simulink model "ProyectoAutomatasSimulink_jona"  (R2015a)
settings: Solver=ode3  SolverMode=SingleTasking  StartTime=0.0  StopTime=inf  FixedStep=dt/10  RelTol=1e-3
values from neighbouring files (symbols this model uses):
  amaxh = 1    [ProyectoAutomatas.m]
  amaxt = 1    [ProyectoAutomatas.m]
  bah = Mh*nh*wposh    (= 69120)    [ProyectoAutomatas.m]
  bat = Mt*nt*wpost    (= 64800)    [ProyectoAutomatas.m]
  bh = beqh*rh^2/Rd^2    (= 28800)    [ProyectoAutomatas.m]
  bt = beqc*rc^2/Rw^2    (= 27000)    [ProyectoAutomatas.m]
  bw = 30*10^3    (= 30000)    [ProyectoAutomatas.m]
  distanciaSegMaxCarro = geometria.xt_max-constSegCarro    [ProyectoAutomatas.m]
  distanciaSegMinCarro = geometria.xt_min+constSegCarro    [ProyectoAutomatas.m]
  dt = 0.01    [ProyectoAutomatas.m]
  g = 9.80665    [ProyectoAutomatas.m]
  Kisah = Mh*wposh^3    (= 17905.2918847)    [ProyectoAutomatas.m]
  Kisat = Mt*wpost^3    (= 9768.17070431)    [ProyectoAutomatas.m]
  Ksah = Mh*nh*wposh^2    (= 49751.6587678)    [ProyectoAutomatas.m]
  Ksat = Mt*nt*wpost^2    (= 35580.2603037)    [ProyectoAutomatas.m]
  Kw = 1800*10^3    (= 1800000)    [ProyectoAutomatas.m]
  l_max_cable = 65    [ProyectoAutomatas.m]
  l_max_max_cable = 66    [ProyectoAutomatas.m]
  l_min_cable = 5    [ProyectoAutomatas.m]
  l_min_min_cable = 4    [ProyectoAutomatas.m]
  lh0 = 5    [ProyectoAutomatas.m]
  longitudSegMaxCable = l_max_cable-constSegCable    (= 60)    [ProyectoAutomatas.m]
  longitudSegMinCable = l_min_cable+constSegCable    (= 10)    [ProyectoAutomatas.m]
  mc = 50000    [ProyectoAutomatas.m]
  Mh = (Jdh+Jmh*rh^2) / (Rd^2)    (= 48014.2222222)    [ProyectoAutomatas.m]
  ml0 = 15000    [ProyectoAutomatas.m]
  mlfull = 65000    [ProyectoAutomatas.m]
  Mt = mc+(Jwc+Jmc*rc^2)/Rw^2    (= 59008)    [ProyectoAutomatas.m]
  na = 3    [ProyectoAutomatas.m]
  rc = 15    [ProyectoAutomatas.m]
  Rd = 0.75    [ProyectoAutomatas.m]
  rh = 30    [ProyectoAutomatas.m]
  Rw = 0.5    [ProyectoAutomatas.m]
  vh0 = 0    [ProyectoAutomatas.m]
  vlx0 = 0    [ProyectoAutomatas.m]
  vly0 = 0    [ProyectoAutomatas.m]
  vmaxh = 3    [ProyectoAutomatas.m]
  vmaxhfull = 1.5    [ProyectoAutomatas.m]
  vmaxhSobrepeso = 0.1    [ProyectoAutomatas.m]
  vmaxt = 4    [ProyectoAutomatas.m]
  vt0 = 0    [ProyectoAutomatas.m]
  xl0 = -30    [ProyectoAutomatas.m]
  xt0 = -30    [ProyectoAutomatas.m]
  xt_max = 50    [ParametrosGUIyTrayectoria.m]    (also in ProyectoAutomatas.m)
  xt_max_max = 51    [ParametrosGUIyTrayectoria.m]    (also in ProyectoAutomatas.m)
  xt_min = -30    [ParametrosGUIyTrayectoria.m]    (also in ProyectoAutomatas.m)
  xt_min_min = -31    [ParametrosGUIyTrayectoria.m]    (also in ProyectoAutomatas.m)
  yl0 = yt0-lh0-ml0*g/Kw    (= 39.9182779167)    [ProyectoAutomatas.m]
  yt0 = 45    [ProyectoAutomatas.m]
libraries: vrlib x1
settings Model: Creator=Garcia Obredor  LastModifiedBy=Maxi Garcia
settings DataIOCC: SignalLoggingSaveFormat=ModelDataLogs
settings OptimizationCC: BlockReduction=off  BooleanDataType=off
settings DebuggingCC: SaveWithParameterizedLinksMsg=none  UnderspecifiedInitializationDetection=Classic  MergeDetectMultiDrivingBlocksExec=none  SignalResolutionControl=TryResolveAllWithWarning  MultiTaskDSMMsg=warning  MultiTaskCondExecSysMsg=none
settings HardwareCC: TargetLongLongMode=on  TargetIntDivRoundTo=Zero  TargetEndianess=LittleEndian  TargetHWDeviceType=MATLAB Host  ProdEqTarget=off

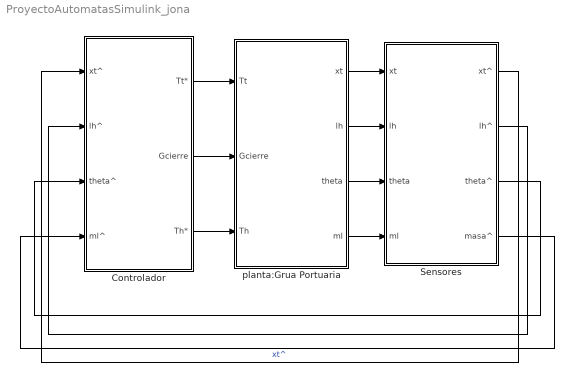
== system ProyectoAutomatasSimulink_jona ==
  Controlador : Subsystem
  Sensores : Subsystem
  planta:Grua Portuaria : Subsystem
  wires:
  planta:Grua Portuaria/4(ml) -> Sensores/4(ml)
  planta:Grua Portuaria/1(xt) -> Sensores/1(xt)
  Controlador/2(Gcierre) -> planta:Grua Portuaria/2(Gcierre)
  planta:Grua Portuaria/3(theta) -> Sensores/3(theta)
  Controlador/3(Th*) -> planta:Grua Portuaria/3(Th)
  Controlador/1(Tt*) -> planta:Grua Portuaria/1(Tt)
  planta:Grua Portuaria/2(lh) -> Sensores/2(lh)
  Sensores/1(xt^) -> Controlador/1(xt^)  "xt^"
  Sensores/2(lh^) -> Controlador/2(lh^)
  Sensores/3(theta^) -> Controlador/3(theta^)
  Sensores/4(masa^) -> Controlador/4(ml^)

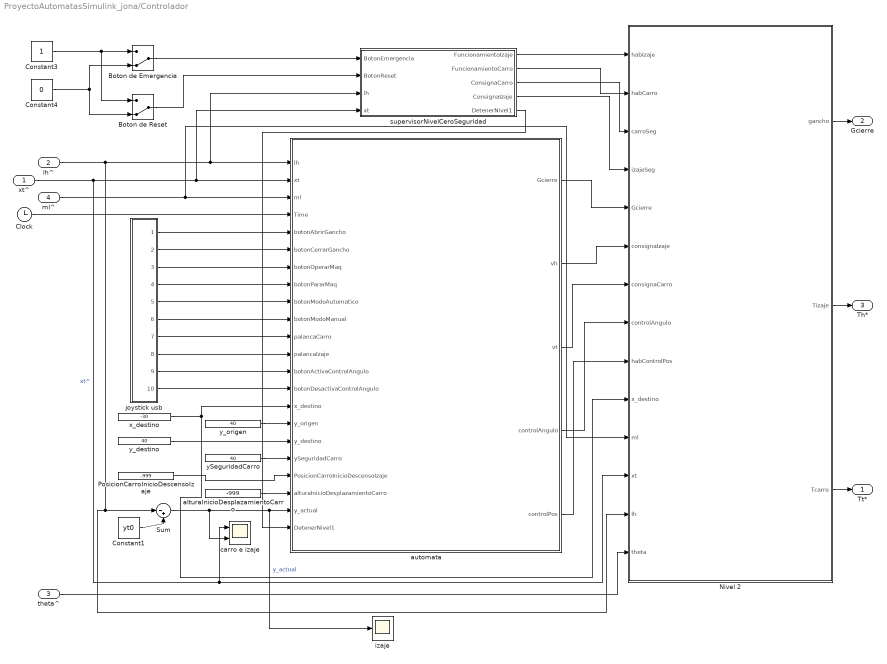
== system ProyectoAutomatasSimulink_jona/Controlador ==
  xt^ : Inport
  lh^ : Inport  Port=2
  theta^ : Inport  Port=3
  ml^ : Inport  Port=4
  Boton de Emergencia : ManualSwitch  CurrentSetting=0
  Boton de Reset : ManualSwitch  CurrentSetting=0
  Clock : Clock
  Constant1 : Constant  Value=yt0
  Constant3 : Constant
  Constant4 : Constant  Value=0
  Nivel 2 : Subsystem
  PosicionCarroInicioDescensoIzaje : Constant  Value=-999
  Sum : Sum  Inputs=|-+
  alturaInicioDesplazamientoCarro : Constant  Value=-999
  automata : Stateflow chart  TreatAsAtomicUnit=on
  carro e izaje : Scope  NumInputPorts=2
      settings: YMin=-38.19374~0.78061  YMax=43.7437~38.75326
  izaje : Scope
      settings: YMin=-36.2214  YMax=37.6181
  joystick usb : Subsystem
  supervisorNivelCeroSeguridad : Stateflow chart  TreatAsAtomicUnit=on
  x_destino : Constant  Value=-30
  ySeguridadCarro : Constant  Value=40
  y_destino : Constant  Value=40
  y_origen : Constant  Value=40
  Tt* : Outport
  Gcierre : Outport  Port=2
  Th* : Outport  Port=3
  wires:
  joystick usb/7(Out8) -> automata/11(palancaCarro)
  joystick usb/1(Out1) -> automata/5(botonAbrirGancho)
  joystick usb/2(Out2) -> automata/6(botonCerrarGancho)
  joystick usb/8(Out9) -> automata/12(palancaIzaje)
  joystick usb/4(Out4) -> automata/8(botonPararMaq)
  joystick usb/5(Out6) -> automata/9(botonModoAutomatico)
  joystick usb/6(Out7) -> automata/10(botonModoManual)
  joystick usb/3(Out3) -> automata/7(botonOperarMaq)
  ySeguridadCarro/1 -> automata/18(ySeguridadCarro)
  PosicionCarroInicioDescensoIzaje/1 -> automata/19(PosicionCarroInicioDescensoIzaje)
  alturaInicioDesplazamientoCarro/1 -> automata/20(alturaInicioDesplazamientoCarro)
  x_destino/1 -> Nivel 2/10(x_destino), automata/15(x_destino)
  Constant1/1 -> Sum/2
  y_destino/1 -> automata/17(y_destino)
  Clock/1 -> automata/4(Time)
  joystick usb/9(Out5) -> automata/13(botonActivaControlAngulo)
  joystick usb/10(Out10) -> automata/14(botonDesactivaControlAngulo)
  Constant3/1 -> Boton de Emergencia/1, Boton de Reset/1
  Constant4/1 -> Boton de Emergencia/2, Boton de Reset/2
  Boton de Reset/1 -> supervisorNivelCeroSeguridad/2(BotonReset)
  Boton de Emergencia/1 -> supervisorNivelCeroSeguridad/1(BotonEmergencia)
  lh^/1 -> automata/1(lh), supervisorNivelCeroSeguridad/3(lh), Sum/1, Nivel 2/13(lh)
  ml^/1 -> automata/3(ml), Nivel 2/11(ml)
  y_origen/1 -> automata/16(y_origen)
  supervisorNivelCeroSeguridad/5(DetenerNivel1) -> automata/22(DetenerNivel1)
  supervisorNivelCeroSeguridad/1(FuncionamientoIzaje) -> Nivel 2/1(habIzaje)
  supervisorNivelCeroSeguridad/2(FuncionamientoCarro) -> Nivel 2/2(habCarro)
  supervisorNivelCeroSeguridad/3(ConsignaCarro) -> Nivel 2/3(carroSeg)
  supervisorNivelCeroSeguridad/4(ConsignaIzaje) -> Nivel 2/4(izajeSeg)
  automata/1(Gcierre) -> Nivel 2/5(Gcierre)
  automata/2(vh) -> Nivel 2/6(consignaIzaje)
  automata/3(vt) -> Nivel 2/7(consignaCarro)
  automata/4(controlAngulo) -> Nivel 2/8(controlAngulo)
  automata/5(controlPos) -> Nivel 2/9(habControlPos)
  theta^/1 -> Nivel 2/14(theta)
  Nivel 2/1(gancho) -> Gcierre/1
  Nivel 2/2(Tizaje) -> Th*/1
  Nivel 2/3(Tcarro) -> Tt*/1
  Sum/1 -> carro e izaje/2, izaje/1, automata/21(y_actual)  "y_actual"
  xt^/1 -> automata/2(xt), supervisorNivelCeroSeguridad/4(xt), carro e izaje/1, Nivel 2/12(xt)  "xt^"

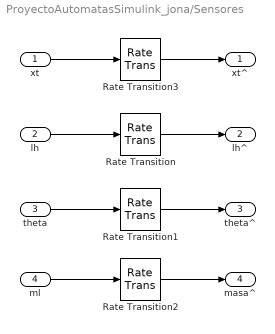
== system ProyectoAutomatasSimulink_jona/Sensores ==
  xt : Inport
  lh : Inport  Port=2
  theta : Inport  Port=3
  ml : Inport  Port=4
  Rate Transition : RateTransition  X0=5  OutPortSampleTime=dt
  Rate Transition1 : RateTransition  OutPortSampleTime=dt
  Rate Transition2 : RateTransition  X0=ml0  OutPortSampleTime=dt
  Rate Transition3 : RateTransition  X0=-30  OutPortSampleTime=dt
  xt^ : Outport
  lh^ : Outport  Port=2
  theta^ : Outport  Port=3
  masa^ : Outport  Port=4
  wires:
  theta/1 -> Rate Transition1/1
  xt/1 -> Rate Transition3/1
  Rate Transition1/1 -> theta^/1
  ml/1 -> Rate Transition2/1
  lh/1 -> Rate Transition/1
  Rate Transition/1 -> lh^/1
  Rate Transition3/1 -> xt^/1
  Rate Transition2/1 -> masa^/1

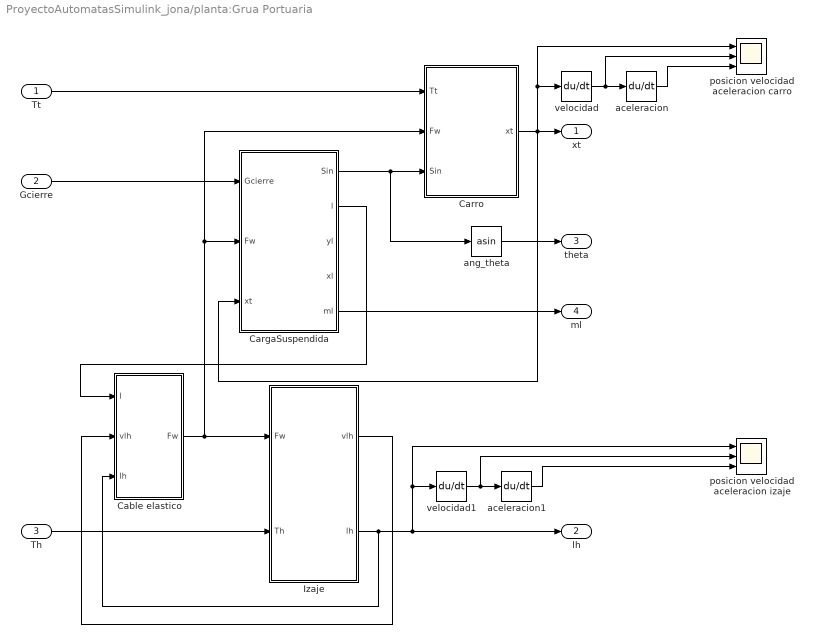
== system ProyectoAutomatasSimulink_jona/planta:Grua Portuaria ==
  Tt : Inport
  Gcierre : Inport  Port=2
  Th : Inport  Port=3
  Cable elastico : Subsystem
  CargaSuspendida : Subsystem
  Carro : Subsystem
  Izaje : Subsystem
  aceleracion : Derivative
  aceleracion1 : Derivative
  ang_theta : Trigonometry  Operator=asin
  posicion velocidad aceleracion carro : Scope  NumInputPorts=3
      settings: ShowLegends=on  YMin=-38.18369~-0.50294~-1.25648  YMax=43.6532~4.52646~1.25794  SaveName=ScopeData5
  posicion velocidad aceleracion izaje : Scope  NumInputPorts=3
      settings: ShowLegends=on  YMin=6.24674~-3.39473~-0.87987  YMax=44.21939~0.40083~1.32498  SaveName=ScopeData6
  velocidad : Derivative
  velocidad1 : Derivative
  xt : Outport
  lh : Outport  Port=2
  theta : Outport  Port=3
  ml : Outport  Port=4
  wires:
  Izaje/1(vlh) -> Cable elastico/2(vlh)
  CargaSuspendida/1(Sin) -> Carro/3(Sin), ang_theta/1
  Th/1 -> Izaje/2(Th)
  Carro/1(xt) -> velocidad/1, posicion velocidad aceleracion carro/1, xt/1, CargaSuspendida/3(xt)
  Gcierre/1 -> CargaSuspendida/1(Gcierre)
  Tt/1 -> Carro/1(Tt)
  CargaSuspendida/2(l) -> Cable elastico/1(l)
  Cable elastico/1(Fw) -> Izaje/1(Fw), Carro/2(Fw), CargaSuspendida/2(Fw)
  ang_theta/1 -> theta/1
  CargaSuspendida/5(ml) -> ml/1
  velocidad/1 -> aceleracion/1, posicion velocidad aceleracion carro/2
  aceleracion/1 -> posicion velocidad aceleracion carro/3
  velocidad1/1 -> aceleracion1/1, posicion velocidad aceleracion izaje/2
  aceleracion1/1 -> posicion velocidad aceleracion izaje/3
  Izaje/2(lh) -> lh/1, velocidad1/1, posicion velocidad aceleracion izaje/1, Cable elastico/3(lh)

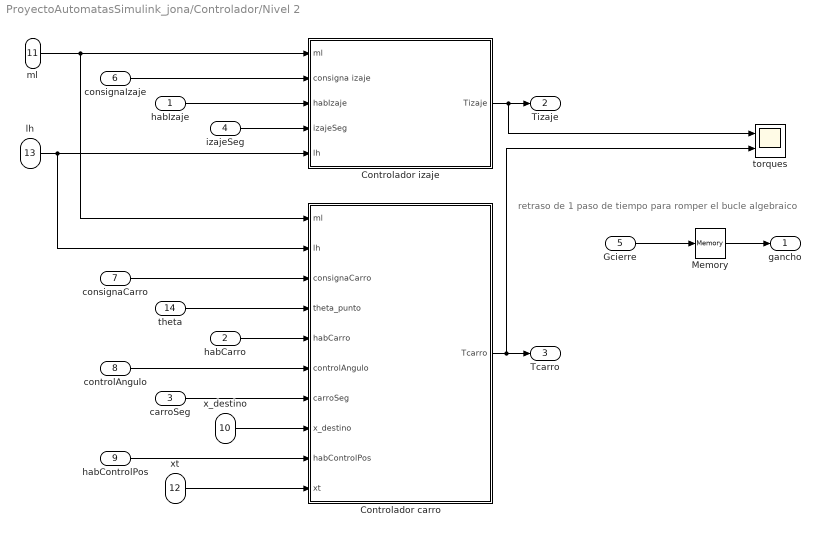
== system ProyectoAutomatasSimulink_jona/Controlador/Nivel 2 ==
  note: retraso de 1 paso de tiempo para romper el bucle algebraico
  habIzaje : Inport
  habCarro : Inport  Port=2
  carroSeg : Inport  Port=3
  izajeSeg : Inport  Port=4
  Gcierre : Inport  Port=5
  consignaIzaje : Inport  Port=6
  consignaCarro : Inport  Port=7
  controlAngulo : Inport  Port=8
  habControlPos : Inport  Port=9
  x_destino : Inport  Port=10
  ml : Inport  Port=11
  xt : Inport  Port=12
  lh : Inport  Port=13
  theta : Inport  Port=14
  Controlador carro : Subsystem
  Controlador izaje : Subsystem
  Memory : Memory
  torques : Scope  NumInputPorts=2
      settings: ShowLegends=on  YMin=-8301.97836~-5  YMax=6865.80026~5
  gancho : Outport
  Tizaje : Outport  Port=2
  Tcarro : Outport  Port=3
  wires:
  Memory/1 -> gancho/1
  Gcierre/1 -> Memory/1
  ml/1 -> Controlador carro/1(ml), Controlador izaje/1(ml)
  lh/1 -> Controlador carro/2(lh), Controlador izaje/5(lh)
  consignaIzaje/1 -> Controlador izaje/2(consigna izaje)
  habIzaje/1 -> Controlador izaje/3(habIzaje)
  izajeSeg/1 -> Controlador izaje/4(izajeSeg)
  Controlador izaje/1(Tizaje) -> torques/1, Tizaje/1
  consignaCarro/1 -> Controlador carro/3(consignaCarro)
  theta/1 -> Controlador carro/4(theta_punto)
  habCarro/1 -> Controlador carro/5(habCarro)
  controlAngulo/1 -> Controlador carro/6(controlAngulo)
  carroSeg/1 -> Controlador carro/7(carroSeg)
  x_destino/1 -> Controlador carro/8(x_destino)
  habControlPos/1 -> Controlador carro/9(habControlPos)
  xt/1 -> Controlador carro/10(xt)
  Controlador carro/1(Tcarro) -> Tcarro/1, torques/2

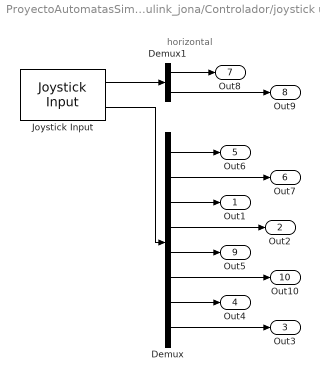
== system ProyectoAutomatasSimulink_jona/Controlador/joystick usb ==
  note: horizontal
  Demux : Demux  Outputs=8
  Demux1 : Demux  Outputs=2
  Joystick Input : vrlib/Joystick Input  joyid=1  adjustports=on  forcefeed=off
  Out1 : Outport
  Out2 : Outport  Port=2
  Out3 : Outport  Port=3
  Out4 : Outport  Port=4
  Out6 : Outport  Port=5
  Out7 : Outport  Port=6
  Out8 : Outport  Port=7
  Out9 : Outport  Port=8
  Out5 : Outport  Port=9
  Out10 : Outport  Port=10
  wires:
  Demux/8 -> Out3/1
  Demux/1 -> Out6/1
  Joystick Input/2 -> Demux/1
  Demux/2 -> Out7/1
  Joystick Input/1 -> Demux1/1
  Demux/7 -> Out4/1
  Demux1/1 -> Out8/1
  Demux1/2 -> Out9/1
  Demux/4 -> Out2/1
  Demux/3 -> Out1/1
  Demux/5 -> Out5/1
  Demux/6 -> Out10/1

== system ProyectoAutomatasSimulink_jona/planta:Grua Portuaria/Cable elastico ==
  l : Inport
  vlh : Inport  Port=2
  lh : Inport  Port=3
  Derivative : Derivative
  Kw : Gain  Gain=Kw
  Sum : Sum  Inputs=|+-
  Sum1 : Sum  Inputs=|-+
  Sum2 : Sum  Inputs=|++
  bw : Gain  Gain=bw
  Fw : Outport
  wires:
  l/1 -> Derivative/1, Sum1/2
  Derivative/1 -> Sum/1
  vlh/1 -> Sum/2
  Sum1/1 -> Kw/1
  Sum/1 -> bw/1
  Kw/1 -> Sum2/1
  bw/1 -> Sum2/2
  Sum2/1 -> Fw/1
  lh/1 -> Sum1/1

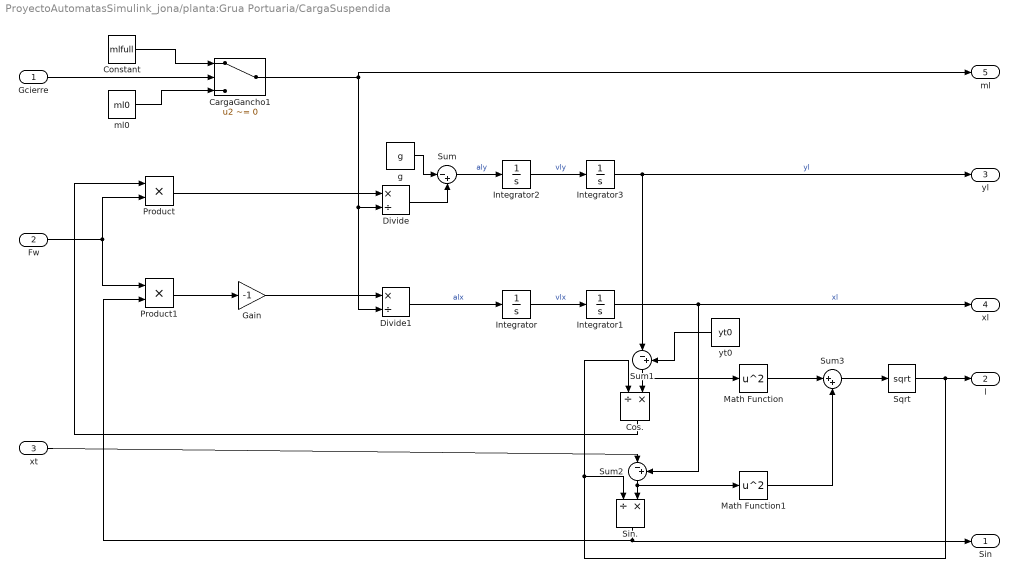
== system ProyectoAutomatasSimulink_jona/planta:Grua Portuaria/CargaSuspendida ==
  Gcierre : Inport
  Fw : Inport  Port=2
  xt : Inport  Port=3
  CargaGancho1 : Switch  Criteria=u2 ~= 0  Threshold=0.5
  Constant : Constant  Value=mlfull
  Cos. : Product  Inputs=/*
  Divide : Product  Inputs=*/
  Divide1 : Product  Inputs=*/
  Gain : Gain  Gain=-1
  Integrator : Integrator  InitialCondition=vlx0
  Integrator1 : Integrator  InitialCondition=xl0
  Integrator2 : Integrator  InitialCondition=vly0
  Integrator3 : Integrator  InitialCondition=yl0
  Math Function : Math  Operator=square  SaturateOnIntegerOverflow=on
  Math Function1 : Math  Operator=square  SaturateOnIntegerOverflow=on
  Product : Product
  Product1 : Product
  Sin. : Product  Inputs=/*
  Sqrt : Sqrt  SaturateOnIntegerOverflow=on
  Sum : Sum  Inputs=|-+
  Sum1 : Sum  Inputs=|-+
  Sum2 : Sum  Inputs=|-+
  Sum3 : Sum  Inputs=|++
  g : Constant  Value=g
  "ml0 " : Constant  Value=ml0
  yt0 : Constant  Value=yt0
  Sin : Outport
  l : Outport  Port=2
  yl : Outport  Port=3
  xl : Outport  Port=4
  ml : Outport  Port=5
  wires:
  CargaGancho1/1 -> ml/1, Divide/2, Divide1/2
  Gcierre/1 -> CargaGancho1/2
  Fw/1 -> Product1/1, Product/2
  Product/1 -> Divide/1
  Product1/1 -> Gain/1
  Gain/1 -> Divide1/1
  Divide/1 -> Sum/2
  g/1 -> Sum/1
  Integrator/1 -> Integrator1/1  "vlx"
  Integrator1/1 -> xl/1, Sum2/2  "xl"
  Integrator2/1 -> Integrator3/1  "vly"
  Sum1/1 -> Cos./2, Math Function/1
  yt0/1 -> Sum1/2
  Integrator3/1 -> yl/1, Sum1/1  "yl"
  Cos./1 -> Product/1
  Sum2/1 -> Math Function1/1, Sin./2
  xt/1 -> Sum2/1
  Sin./1 -> Sin/1, Product1/2
  Math Function/1 -> Sum3/1
  Math Function1/1 -> Sum3/2
  Sum3/1 -> Sqrt/1
  Constant/1 -> CargaGancho1/1
  "ml0 "/1 -> CargaGancho1/3
  Sqrt/1 -> Cos./1, Sin./1, l/1
  Sum/1 -> Integrator2/1  "aly"
  Divide1/1 -> Integrator/1  "alx"

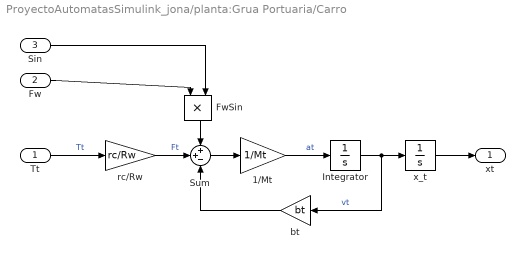
== system ProyectoAutomatasSimulink_jona/planta:Grua Portuaria/Carro ==
  Tt : Inport
  Fw : Inport  Port=2
  Sin : Inport  Port=3
  1/Mt : Gain  Gain=1/Mt
  FwSin : Product
  Integrator : Integrator  InitialCondition=vt0
  Sum : Sum  Inputs=++-
  bt : Gain  Gain=bt
  rc/Rw : Gain  Gain=rc/Rw
  x_t : Integrator  InitialCondition=xt0
  xt : Outport
  wires:
  x_t/1 -> xt/1
  rc/Rw/1 -> Sum/2  "Ft"
  Tt/1 -> rc/Rw/1  "Tt"
  1/Mt/1 -> Integrator/1  "at"
  bt/1 -> Sum/3
  Sum/1 -> 1/Mt/1
  Integrator/1 -> x_t/1, bt/1  "vt"
  Sin/1 -> FwSin/2
  FwSin/1 -> Sum/1
  Fw/1 -> FwSin/1

== system ProyectoAutomatasSimulink_jona/planta:Grua Portuaria/Izaje ==
  Fw : Inport
  Th : Inport  Port=2
  "-rh/Rd\t" : Gain  Gain=-rh/Rd
  1/Mh : Gain  Gain=1/Mh
  Integrator : Integrator  InitialCondition=vh0
  Sum : Sum  Inputs=+--
  bh : Gain  Gain=bh
  l_h : Integrator  InitialCondition=lh0
  vlh : Outport
  lh : Outport  Port=2
  wires:
  l_h/1 -> lh/1
  "-rh/Rd\t"/1 -> Sum/2  "Fh"
  Th/1 -> "-rh/Rd\t"/1  "Th"
  1/Mh/1 -> Integrator/1  "ah"
  bh/1 -> Sum/3
  Sum/1 -> 1/Mh/1
  Integrator/1 -> l_h/1, vlh/1, bh/1  "vh"
  Fw/1 -> Sum/1

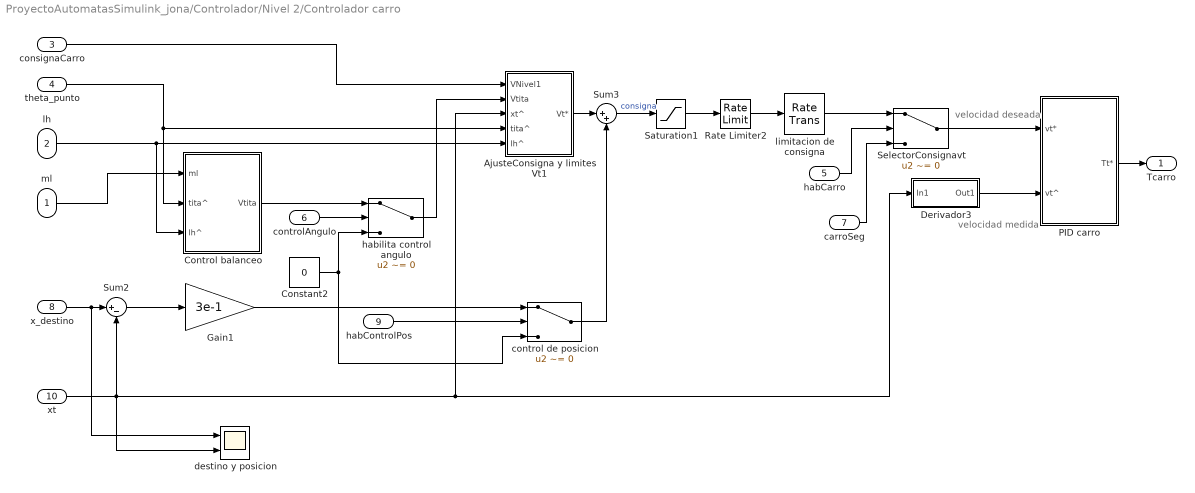
== system ProyectoAutomatasSimulink_jona/Controlador/Nivel 2/Controlador carro ==
  note: velocidad deseada
  note: velocidad medida
  ml : Inport
  lh : Inport  Port=2
  consignaCarro : Inport  Port=3
  theta_punto : Inport  Port=4
  habCarro : Inport  Port=5
  controlAngulo : Inport  Port=6
  carroSeg : Inport  Port=7
  x_destino : Inport  Port=8
  habControlPos : Inport  Port=9
  xt : Inport  Port=10
  AjusteConsigna y limites Vt1 : Subsystem
  Constant2 : Constant  Value=0
  Control balanceo : Subsystem
  Derivador3 : Subsystem
  Gain1 : Gain  Gain=3e-1
  PID carro : Subsystem
  Rate Limiter2 : RateLimiter  RisingSlewLimit=amaxt  FallingSlewLimit=-amaxt  SampleTimeMode=inherited
  Saturation1 : Saturate  UpperLimit=vmaxt  LowerLimit=-vmaxt
  SelectorConsignavt : Switch  Criteria=u2 ~= 0  Threshold=0.5
  Sum2 : Sum  Inputs=|+-
  Sum3 : Sum  Inputs=|++
  control de posicion : Switch  Criteria=u2 ~= 0  Threshold=0.5
  destino y posicion : Scope  NumInputPorts=2
      settings: YMin=-37.93488~-5  YMax=41.10237~5
  habilita control angulo : Switch  Criteria=u2 ~= 0  Threshold=0.5
  limitacion de consigna : RateTransition  OutPortSampleTime=dt
  Tcarro : Outport
  wires:
  Gain1/1 -> control de posicion/1
  habilita control angulo/1 -> AjusteConsigna y limites Vt1/2(Vtita)
  PID carro/1(Tt*) -> Tcarro/1
  control de posicion/1 -> Sum3/2
  habControlPos/1 -> control de posicion/2
  AjusteConsigna y limites Vt1/1(Vt*) -> Sum3/1
  Rate Limiter2/1 -> limitacion de consigna/1
  Saturation1/1 -> Rate Limiter2/1
  Sum3/1 -> Saturation1/1  "consigna"
  Sum2/1 -> Gain1/1
  Constant2/1 -> control de posicion/3, habilita control angulo/3
  controlAngulo/1 -> habilita control angulo/2
  Derivador3/1(Out1) -> PID carro/2(vt^)
  habCarro/1 -> SelectorConsignavt/2
  SelectorConsignavt/1 -> PID carro/1(vt*)
  theta_punto/1 -> Control balanceo/2(tita^), AjusteConsigna y limites Vt1/4(tita^)
  consignaCarro/1 -> AjusteConsigna y limites Vt1/1(VNivel1)
  carroSeg/1 -> SelectorConsignavt/3
  xt/1 -> destino y posicion/2, Sum2/2, AjusteConsigna y limites Vt1/3(xt^), Derivador3/1(In1)
  x_destino/1 -> Sum2/1, destino y posicion/1
  lh/1 -> Control balanceo/3(lh^), AjusteConsigna y limites Vt1/5(lh^)
  ml/1 -> Control balanceo/1(ml)
  Control balanceo/1(Vtita) -> habilita control angulo/1
  limitacion de consigna/1 -> SelectorConsignavt/1

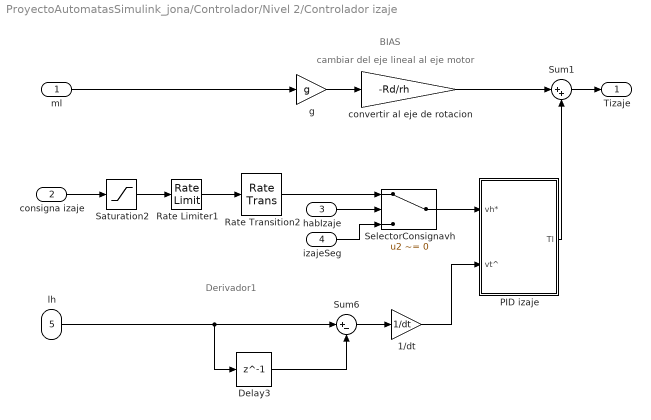
== system ProyectoAutomatasSimulink_jona/Controlador/Nivel 2/Controlador izaje ==
  note: Derivador1
  note: cambiar del eje lineal al eje motor
  note: BIAS
  ml : Inport
  consigna izaje : Inport  Port=2
  habIzaje : Inport  Port=3
  izajeSeg : Inport  Port=4
  lh : Inport  Port=5
  1/dt : Gain  Gain=1/dt
  Delay3 : Delay  DelayLength=1  InitialCondition=5  SampleTime=dt
  PID izaje : Subsystem
  Rate Limiter1 : RateLimiter  RisingSlewLimit=amaxh  FallingSlewLimit=-amaxh  SampleTimeMode=inherited
  Rate Transition2 : RateTransition  X0=5  OutPortSampleTime=dt
  Saturation2 : Saturate  UpperLimit=vmaxh  LowerLimit=-vmaxh
  SelectorConsignavh : Switch  Criteria=u2 ~= 0  Threshold=0.5
  Sum1 : Sum  Inputs=|++
  Sum6 : Sum  Inputs=|+-
  convertir al eje de rotacion : Gain  Gain=-Rd/rh
  g : Gain  Gain=g
  Tizaje : Outport
  wires:
  PID izaje/1(Tl) -> Sum1/2
  SelectorConsignavh/1 -> PID izaje/1(vh*)
  Rate Transition2/1 -> SelectorConsignavh/1
  Rate Limiter1/1 -> Rate Transition2/1
  habIzaje/1 -> SelectorConsignavh/2
  consigna izaje/1 -> Saturation2/1
  1/dt/1 -> PID izaje/2(vt^)
  Saturation2/1 -> Rate Limiter1/1
  convertir al eje de rotacion/1 -> Sum1/1
  g/1 -> convertir al eje de rotacion/1
  Sum1/1 -> Tizaje/1
  izajeSeg/1 -> SelectorConsignavh/3
  ml/1 -> g/1
  Sum6/1 -> 1/dt/1
  Delay3/1 -> Sum6/2
  lh/1 -> Delay3/1, Sum6/1

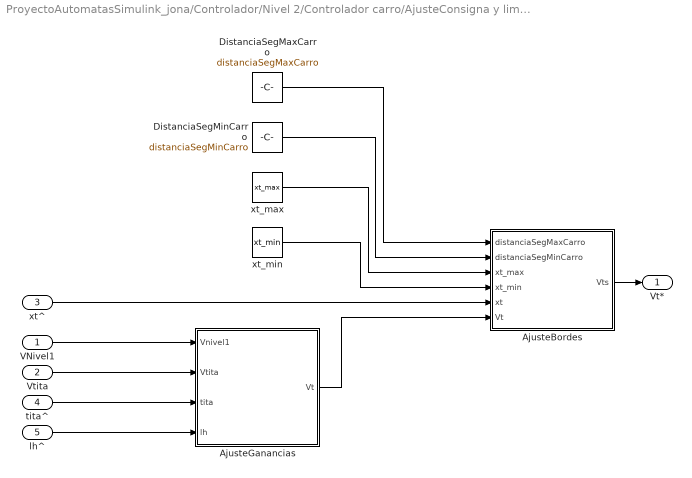
== system ProyectoAutomatasSimulink_jona/Controlador/Nivel 2/Controlador carro/AjusteConsigna y limites Vt1 ==
  VNivel1 : Inport
  Vtita : Inport  Port=2
  xt^ : Inport  Port=3
  tita^ : Inport  Port=4
  lh^ : Inport  Port=5
  AjusteBordes : MATLAB Function  TreatAsAtomicUnit=on
  AjusteGanancias : MATLAB Function  TreatAsAtomicUnit=on
  DistanciaSegMaxCarro : Constant  Value=distanciaSegMaxCarro
  DistanciaSegMinCarro : Constant  Value=distanciaSegMinCarro
  xt_max : Constant  Value=xt_max
  xt_min : Constant  Value=xt_min
  Vt* : Outport
  wires:
  AjusteGanancias/1(Vt) -> AjusteBordes/6(Vt)
  Vtita/1 -> AjusteGanancias/2(Vtita)
  VNivel1/1 -> AjusteGanancias/1(Vnivel1)
  xt_min/1 -> AjusteBordes/4(xt_min)
  xt_max/1 -> AjusteBordes/3(xt_max)
  DistanciaSegMinCarro/1 -> AjusteBordes/2(distanciaSegMinCarro)
  DistanciaSegMaxCarro/1 -> AjusteBordes/1(distanciaSegMaxCarro)
  xt^/1 -> AjusteBordes/5(xt)
  AjusteBordes/1(Vts) -> Vt*/1
  tita^/1 -> AjusteGanancias/3(tita)
  lh^/1 -> AjusteGanancias/4(lh)

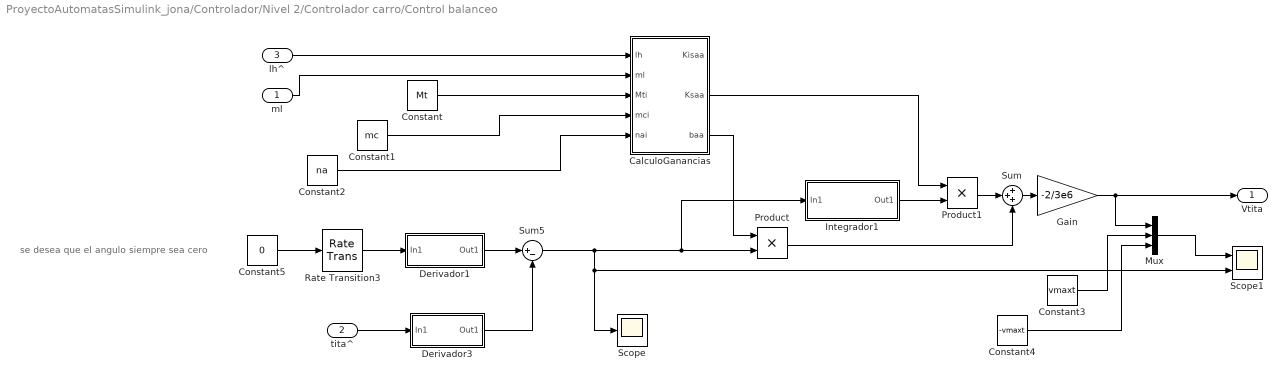
== system ProyectoAutomatasSimulink_jona/Controlador/Nivel 2/Controlador carro/Control balanceo ==
  note: se desea que el angulo siempre sea cero
  ml : Inport
  tita^ : Inport  Port=2
  lh^ : Inport  Port=3
  CalculoGanancias : MATLAB Function  TreatAsAtomicUnit=on
  Constant : Constant  Value=Mt
  Constant1 : Constant  Value=mc
  Constant2 : Constant  Value=na
  Constant3 : Constant  Value=vmaxt
  Constant4 : Constant  Value=-vmaxt
  Constant5 : Constant  Value=0
  Derivador1 : Subsystem
  Derivador3 : Subsystem
  Gain : Gain  Gain=-2/3e6
  Integrador1 : Subsystem
  Mux : Mux  Inputs=3
  Product : Product
  Product1 : Product
  Rate Transition3 : RateTransition  OutPortSampleTime=dt
  Scope : Scope
      settings: YMin=-1.2  YMax=0.7  SaveName=ScopeData9
  Scope1 : Scope  NumInputPorts=2
      settings: YMin=-8.11572~-0.13558  YMax=12.0677~0.14447
  Sum : Sum  Inputs=+++
  Sum5 : Sum  Inputs=|+-
  Vtita : Outport
  wires:
  Sum5/1 -> Scope/1, Scope1/2, Integrador1/1(In1), Product/2
  Derivador3/1(Out1) -> Sum5/2
  Derivador1/1(Out1) -> Sum5/1
  Constant2/1 -> CalculoGanancias/5(nai)
  Constant1/1 -> CalculoGanancias/4(mci)
  Constant/1 -> CalculoGanancias/3(Mti)
  ml/1 -> CalculoGanancias/2(ml)
  CalculoGanancias/2(Ksaa) -> Product1/1
  CalculoGanancias/3(baa) -> Product/1
  tita^/1 -> Derivador3/1(In1)
  Product1/1 -> Sum/2
  Integrador1/1(Out1) -> Product1/2
  Product/1 -> Sum/3
  lh^/1 -> CalculoGanancias/1(lh)
  Rate Transition3/1 -> Derivador1/1(In1)
  Mux/1 -> Scope1/1
  Gain/1 -> Vtita/1, Mux/1
  Constant3/1 -> Mux/2
  Constant4/1 -> Mux/3
  Constant5/1 -> Rate Transition3/1
  Sum/1 -> Gain/1

== system ProyectoAutomatasSimulink_jona/Controlador/Nivel 2/Controlador carro/Derivador3 ==
  In1 : Inport
  1/dt : Gain  Gain=1/dt
  Delay3 : Delay  DelayLength=1  InitialCondition=-30  SampleTime=dt
  Sum6 : Sum  Inputs=|+-
  Out1 : Outport
  wires:
  In1/1 -> Delay3/1, Sum6/1
  Delay3/1 -> Sum6/2
  Sum6/1 -> 1/dt/1
  1/dt/1 -> Out1/1

== system ProyectoAutomatasSimulink_jona/Controlador/Nivel 2/Controlador carro/PID carro ==
  vt* : Inport
  vt^ : Inport  Port=2
  PID discreto : Subsystem
  Sum5 : Sum  Inputs=|+-
  error de velocidad carro : Scope
      settings: ShowLegends=on  YMin=-0.07409  YMax=0.05442  SaveName=ScopeData4
  Tt* : Outport
  wires:
  vt*/1 -> Sum5/1
  vt^/1 -> Sum5/2
  Sum5/1 -> error de velocidad carro/1, PID discreto/1(error velocidad)
  PID discreto/1(Out1) -> Tt*/1

== system ProyectoAutomatasSimulink_jona/Controlador/Nivel 2/Controlador izaje/PID izaje ==
  vh* : Inport
  vt^ : Inport  Port=2
  PID Discreto : Subsystem
  Sum5 : Sum  Inputs=|+-
  Tl : Outport
  wires:
  vh*/1 -> Sum5/1
  vt^/1 -> Sum5/2
  Sum5/1 -> PID Discreto/1(error)
  PID Discreto/1(Out1) -> Tl/1

== system ProyectoAutomatasSimulink_jona/Controlador/Nivel 2/Controlador carro/Control balanceo/Derivador1 ==
  In1 : Inport
  1/dt : Gain  Gain=1/dt
  Delay3 : Delay  DelayLength=1  InitialCondition=0  SampleTime=dt
  Sum6 : Sum  Inputs=|+-
  Out1 : Outport
  wires:
  In1/1 -> Delay3/1, Sum6/1
  Delay3/1 -> Sum6/2
  Sum6/1 -> 1/dt/1
  1/dt/1 -> Out1/1

== system ProyectoAutomatasSimulink_jona/Controlador/Nivel 2/Controlador carro/Control balanceo/Derivador3 ==
  In1 : Inport
  1/dt : Gain  Gain=1/dt
  Delay3 : Delay  DelayLength=1  InitialCondition=0  SampleTime=dt
  Sum6 : Sum  Inputs=|+-
  Out1 : Outport
  wires:
  In1/1 -> Delay3/1, Sum6/1
  Delay3/1 -> Sum6/2
  Sum6/1 -> 1/dt/1
  1/dt/1 -> Out1/1

== system ProyectoAutomatasSimulink_jona/Controlador/Nivel 2/Controlador carro/Control balanceo/Integrador1 ==
  In1 : Inport
  Delay3 : Delay  DelayLength=1  SampleTime=dt
  Sum6 : Sum  Inputs=|++
  dt : Gain  Gain=dt
  Out1 : Outport
  wires:
  Delay3/1 -> Sum6/2
  Sum6/1 -> Out1/1, Delay3/1
  dt/1 -> Sum6/1
  In1/1 -> dt/1

== system ProyectoAutomatasSimulink_jona/Controlador/Nivel 2/Controlador carro/PID carro/PID discreto ==
  note: Integrador1
  error velocidad : Inport
  Delay3 : Delay  DelayLength=1  SampleTime=dt
  Integrador : Subsystem
  Kisat : Gain  Gain=Kisat
  Ksat : Gain  Gain=Ksat
  Sum : Sum  Inputs=+++
  Sum6 : Sum  Inputs=|++
  bat : Gain  Gain=bat
  dt : Gain  Gain=dt
  Out1 : Outport
  wires:
  bat/1 -> Sum/3
  Ksat/1 -> Sum/2
  Kisat/1 -> Sum/1
  Sum/1 -> Out1/1
  Integrador/1(Out1) -> Kisat/1
  Sum6/1 -> Integrador/1(In1), Ksat/1, Delay3/1
  error velocidad/1 -> dt/1, bat/1
  dt/1 -> Sum6/1
  Delay3/1 -> Sum6/2

== system ProyectoAutomatasSimulink_jona/Controlador/Nivel 2/Controlador izaje/PID izaje/PID Discreto ==
  error : Inport
  Integrador : Subsystem
  Integrador1 : Subsystem
  Kisah : Gain  Gain=Kisah
  Ksah : Gain  Gain=Ksah
  Sum : Sum  Inputs=+++
  bah : Gain  Gain=bah
  Out1 : Outport
  wires:
  error/1 -> Integrador1/1(In1), bah/1
  Kisah/1 -> Sum/1
  bah/1 -> Sum/3
  Sum/1 -> Out1/1
  Integrador/1(Out1) -> Kisah/1
  Integrador1/1(Out1) -> Integrador/1(In1), Ksah/1
  Ksah/1 -> Sum/2

== system ProyectoAutomatasSimulink_jona/Controlador/Nivel 2/Controlador carro/PID carro/PID discreto/Integrador ==
  In1 : Inport
  Delay3 : Delay  DelayLength=1  SampleTime=dt
  Sum6 : Sum  Inputs=|++
  dt : Gain  Gain=dt
  Out1 : Outport
  wires:
  Delay3/1 -> Sum6/2
  Sum6/1 -> Out1/1, Delay3/1
  dt/1 -> Sum6/1
  In1/1 -> dt/1

== system ProyectoAutomatasSimulink_jona/Controlador/Nivel 2/Controlador izaje/PID izaje/PID Discreto/Integrador ==
  In1 : Inport
  Delay3 : Delay  DelayLength=1  SampleTime=dt
  Sum6 : Sum  Inputs=|++
  dt : Gain  Gain=dt
  Out1 : Outport
  wires:
  Delay3/1 -> Sum6/2
  Sum6/1 -> Out1/1, Delay3/1
  dt/1 -> Sum6/1
  In1/1 -> dt/1

== system ProyectoAutomatasSimulink_jona/Controlador/Nivel 2/Controlador izaje/PID izaje/PID Discreto/Integrador1 ==
  In1 : Inport
  Delay3 : Delay  DelayLength=1  SampleTime=dt
  Sum6 : Sum  Inputs=|++
  dt : Gain  Gain=dt
  Out1 : Outport
  wires:
  Delay3/1 -> Sum6/2
  Sum6/1 -> Out1/1, Delay3/1
  dt/1 -> Sum6/1
  In1/1 -> dt/1

== stateflow chart ProyectoAutomatasSimulink_jona/Controlador/supervisorNivelCeroSeguridad ==
  state FuncionamientoNormal
    during:
    FuncionamientoIzaje=1;
    FuncionamientoCarro=1;
    DetenerNivel1=0;
  state RestaurarFuncionamiento
    entry:
    IzajeListo=0;
    CarroListo=0;
    state RestaurarCarro [parallel]
      settings: executionOrder=2
      state DetenerCarro
        during:
        if (xt>=xt_max_max || xt<=xt_min_min)
        FuncionamientoCarro=0;
        ConsignaCarro=0;
        end
      state RegresarCarroNormalidad
        during:
        DetenerNivel1=1;
        FuncionamientoCarro=0;
        if xt>xt_max
        ConsignaCarro=-vmaxt/10;
        elseif xt<xt_min
        ConsignaCarro=vmaxt/10;
        end
      state CarroDentroLimites
        during:
        CarroListo=1;
        ConsignaCarro=0;
      (default) -> DetenerCarro
      DetenerCarro -> RegresarCarroNormalidad : [BotonReset==1]
      RegresarCarroNormalidad -> CarroDentroLimites : [xt<=xt_max && xt>=xt_min]
    state RestaurarIzaje [parallel]
      settings: executionOrder=1
      state DetenerIzaje
        during:
        if (lh>l_max_max_cable || lh<l_min_min_cable)
        FuncionamientoIzaje=0;
        ConsignaIzaje=0;
        end
      state RegresarIzajeNormalidad
        during:
        DetenerNivel1=1;
        FuncionamientoIzaje=0;
        if lh>l_max_cable
        ConsignaIzaje=-vmaxh/10;
        elseif lh<l_min_cable
        ConsignaIzaje=vmaxh/10;
        end
      state IzajeDentroLimites
        during:
        IzajeListo=1;
        ConsignaIzaje=0;
      (default) -> DetenerIzaje
      DetenerIzaje -> RegresarIzajeNormalidad : [BotonReset==1]
      RegresarIzajeNormalidad -> IzajeDentroLimites : [lh<=l_max_cable && lh>=l_min_cable]
  state Emergencia
    during:
    FuncionamientoIzaje=0;
    FuncionamientoCarro=0;
    ConsignaIzaje=0;
    ConsignaCarro=0;
    DetenerNivel1=1;
  FuncionamientoNormal -> RestaurarFuncionamiento [order 2] : [lh>l_max_max_cable || lh<l_min_min_cable || xt>=xt_max_max || xt<=xt_min_min]
  RestaurarFuncionamiento -> FuncionamientoNormal [order 2] : [BotonReset==1 && IzajeListo==1 && CarroListo==1]
  (default) -> FuncionamientoNormal
  Emergencia -> FuncionamientoNormal : [BotonEmergencia==0 && BotonReset==1]
  FuncionamientoNormal -> Emergencia [order 1] : [BotonEmergencia==1]
  RestaurarFuncionamiento -> Emergencia [order 1] : [BotonEmergencia==1]
  data: FuncionamientoIzaje output; FuncionamientoCarro output; BotonEmergencia input; BotonReset input; lh input; xt input; xt_max_max parameter; xt_min_min parameter; l_min_min_cable parameter; l_max_max_cable parameter; ConsignaCarro output; ConsignaIzaje output; DetenerNivel1 output; vmaxt parameter; vmaxh parameter; IzajeListo local; CarroListo local; xt_max parameter; xt_min parameter; l_max_cable parameter; l_min_cable parameter

== matlab function ProyectoAutomatasSimulink_jona/Controlador/Nivel 2/Controlador carro/AjusteConsigna y limites Vt1/AjusteBordes ==
  data: distanciaSegMaxCarro input; distanciaSegMinCarro input; xt_max input; xt_min input; xt input; Vt input; Vts output
function Vts = fcn(distanciaSegMaxCarro,distanciaSegMinCarro,xt_max,xt_min,xt,Vt)

if  xt<distanciaSegMinCarro && Vt<0
    m=1/(distanciaSegMinCarro-xt_min);
    yRecta=m*(xt-xt_min);
    if yRecta<0
        yRecta=0;
    end
    Vt=yRecta*Vt;
elseif xt>distanciaSegMaxCarro &&Vt>0
    m=1/(distanciaSegMaxCarro-xt_max);
    yRecta=m*(xt-xt_max);
    if yRecta<0
        yRecta=0;
    end
    Vt=yRecta*Vt;
end
Vts=Vt;

== matlab function ProyectoAutomatasSimulink_jona/Controlador/Nivel 2/Controlador carro/Control balanceo/CalculoGanancias ==
  data: Kisaa output; Ksaa output; baa output; lh input; ml input; Mti input; mci input; nai input
function [Kisaa,Ksaa,baa]= fcn(lh,ml,Mti,mci,nai)

persistent Mt
if isempty(Mt)
   Mt=Mti;
end
persistent mc
if isempty(mc)
   mc=mci;
end
persistent na
if isempty(na)
   na=nai;
end
persistent g
if isempty(g)
   g=9.80665;
end

Ma=(ml+Mt)/(mc+ml)*lh;
wa=(4*(Mt+ml)*Mt*g*lh)^0.5/(2*(Mt+ml))*lh;
wposa=1.6*wa;
baa=Ma*na*wposa;
Ksaa=baa*wposa;
Kisaa=Ksaa*wposa/na;

== matlab function ProyectoAutomatasSimulink_jona/Controlador/Nivel 2/Controlador carro/AjusteConsigna y limites Vt1/AjusteGanancias ==
  data: Vnivel1 input; Vtita input; tita input; Vt output; lh input
function Vt = fcn(Vnivel1,Vtita,tita,lh)

x=abs(tita*180/pi);
if lh>15 %&& x>=.3 
    x0=0;                       %el controlador comienza a trabajar en 1°
    x1=20;                      %el controlador de angulo tiene total preponderancia a los 20°
    m=1/(x1-x0);
    y=m*(x-x0);
    Vt=Vtita*y+Vnivel1*(1-y);
elseif lh<=15 %%|| x<=.3
    x0=0;                       %el controlador comienza a trabajar en 1°
    x1=20;                      %el controlador de angulo tiene total preponderancia a los 20°
    m=1/(x1-x0);
    y=m*(x-x0);
    Vt=Vtita*15+Vnivel1;
else
    Vt=Vnivel1;
end

== stateflow chart ProyectoAutomatasSimulink_jona/Controlador/automata ==
  state automata
    state tableroDeControl [parallel]
      settings: executionOrder=1
      state tableroInactivo
      state tableroActivo
        entry: tiempoTableroActivo = temporalCount(sec);
        during: tiempoTableroActivo = temporalCount(sec);
      tableroActivo -> tableroActivo [order 1] : [botonAbrirGancho || botonCerrarGancho || botonOperarMaq || botonPararMaq || botonModoAutomatico || botonModoManual || palancaCarro || palancaIzaje]
      (default) -> tableroInactivo
      tableroActivo -> tableroInactivo [order 2] : [tiempoTableroActivo>=1]
      tableroInactivo -> tableroActivo : [botonAbrirGancho || botonCerrarGancho || botonOperarMaq || botonPararMaq || botonModoAutomatico || botonModoManual || palancaCarro || palancaIzaje]
    state grua [parallel]
      settings: executionOrder=2
      state maquinaEspera
        entry:
        vt=0;
        vh=0;
        vtPermitida=[0  0];
        vhPermitida=[0 0];
      state maquinaOperando
        state gancho [parallel]
          settings: executionOrder=6
          state Gcerrado
            entry:
            Gcierre=1;
            state pesoPermitido
              entry:
              vhPermitida=[vmaxhfull vmaxhfull];
            state pesoExcedido
              entry:
              vhPermitida=[vmaxhSobrepeso vmaxhSobrepeso];
            (default) -> pesoPermitido
            pesoExcedido -> pesoPermitido : [ml<=mlfull]
            pesoPermitido -> pesoExcedido : [ml>mlfull]
          state Gabierto
            entry:
            Gcierre=0;
            vhPermitida=[vmaxh vmaxh];
          Gabierto -> Gcerrado : [botonCerrarGancho]
          Gcerrado -> Gabierto : [botonAbrirGancho]
          (default) -> Gabierto
        state CalculoSalidas [parallel]
          settings: executionOrder=3
          state ManualAuto
            entry: time0=Time;
            dt=0;
            during:
            dt=Time-time0;
            [vt,vh]=Transferencia(1,dt,vtmanual,vtauto,vhmanual,vhauto);
          state Manual
            entry:
            controlPos =0;
            finOperacion=1;
            during:
            vt=vtmanual;
            vh=vhmanual;
          state AutoManual
            entry: time0=Time;
            dt=0;
            during:
            dt=Time-time0;
            [vt,vh]=Transferencia(-1,dt,vtmanual,vtauto,vhmanual,vhauto);
          state Automatico
            during:
            vt=vtauto;
            vh=vhauto;
          (junction 512) -> ManualAuto [order 1] : [y_actual>y_origen]
          (junction 512) -> Manual [order 2] : [y_actual<y_origen]
          Manual -> (junction 512) : [botonModoAutomatico]
          ManualAuto -> Automatico : [dt>=5]
          AutoManual -> Manual : [dt>=5]
          Automatico -> AutoManual [order 1] : [botonModoManual==1 || in(tableroDeControl.tableroActivo)]
          (default) -> Manual
          Automatico -> Manual [order 2] : [finOperacion]
        state habilitaControlAngulo [parallel]
          settings: executionOrder=5
          state deshabilitado
            entry:
            controlAngulo=0;
          state habilitado
            entry:
            controlAngulo=1;
          (default) -> habilitado
          deshabilitado -> habilitado : [botonActivaControlAngulo]
          habilitado -> deshabilitado : [botonDesactivaControlAngulo]
        state limitesIzaje [parallel]
          settings: executionOrder=1
          state dentroDeLimites
            entry:
            if in(gancho.Gabierto)
            vhPermitida=[vmaxh vmaxh];
            else
            vhPermitida=[vmaxhfull vmaxhfull];
            end
          state cercaLimiteMaximo
            during:
            if in(gancho.Gabierto)
            vhPermitida(1)=rectaDosPuntos(vmaxh,0,longitudSegMaxCable,l_max_cable,lh);
            else
            vhPermitida(1)=rectaDosPuntos(vmaxhfull,0,longitudSegMaxCable,l_max_cable,lh);
            end
          state cercaLimiteMinimo
            during:
            if in(gancho.Gabierto)
            vhPermitida(2)=rectaDosPuntos(vmaxh,0,longitudSegMinCable,l_min_cable,lh);
            else
            vhPermitida(2)=rectaDosPuntos(vmaxhfull,0,longitudSegMinCable,l_min_cable,lh);
            end
            note: el primer elemento de vhPermitida es la velocidad hacia arriba
          (default) -> dentroDeLimites
          cercaLimiteMaximo -> dentroDeLimites : [lh<longitudSegMaxCable]
          dentroDeLimites -> cercaLimiteMaximo [order 1] : [lh>=longitudSegMaxCable]
          dentroDeLimites -> cercaLimiteMinimo [order 2] : [lh<longitudSegMinCable]
          cercaLimiteMinimo -> dentroDeLimites : [lh>=longitudSegMinCable]
        state opAutomatica [parallel]
          settings: executionOrder=4
          state controlMovimientos [parallel]
            settings: executionOrder=1
            state barcoAlMuelle
              state subirIzaje
                en: vhauto=-vhPermitida(2);
              state subirYdesplazarCarro
                en: vtauto=-vmaxt;
              state moverCarro
                en:vhauto=0;
              state bajarYdesplazarCarro
                entry:
                vhauto=vhPermitida(1);
                controlPos =1;
              state bajarCarro
                entry: vtauto=0;
              state parar
                entry: vhauto=0;
                during:
                if temporalCount(sec) >20
                finOperacion=1;
                end
              (default) -> automata.grua.maquinaOperando.opAutomatica.controlMovimientos.barcoAlMuelle.subirIzaje
              automata.grua.maquinaOperando.opAutomatica.controlMovimientos.barcoAlMuelle.subirIzaje -> automata.grua.maquinaOperando.opAutomatica.controlMovimientos.barcoAlMuelle.subirYdesplazarCarro : [y_actual>=alturaInicioDesplazamientoCarro]
              automata.grua.maquinaOperando.opAutomatica.controlMovimientos.barcoAlMuelle.subirYdesplazarCarro -> automata.grua.maquinaOperando.opAutomatica.controlMovimientos.barcoAlMuelle.moverCarro : [y_actual>=ySeguridadCarro-cteAlturaSuperior1]
              automata.grua.maquinaOperando.opAutomatica.controlMovimientos.barcoAlMuelle.moverCarro -> automata.grua.maquinaOperando.opAutomatica.controlMovimientos.barcoAlMuelle.bajarYdesplazarCarro : [xt<PosicionCarroInicioDescensoIzaje+cteDestino]
              automata.grua.maquinaOperando.opAutomatica.controlMovimientos.barcoAlMuelle.bajarYdesplazarCarro -> automata.grua.maquinaOperando.opAutomatica.controlMovimientos.barcoAlMuelle.bajarCarro : [xt<x_destino+cteDestino+cteCarro]
              automata.grua.maquinaOperando.opAutomatica.controlMovimientos.barcoAlMuelle.bajarCarro -> automata.grua.maquinaOperando.opAutomatica.controlMovimientos.barcoAlMuelle.parar : [y_actual<=y_destino+cteAlturaInferior]
            state muelleAlBarco
              state subirIzaje
                en: vhauto=-vhPermitida(2);
              state subirYdesplazarCarro
                en: vtauto=vmaxt;
              state moverCarro
                en: vhauto=0;
              state bajarYdesplazarCarro
                entry:
                vhauto=vhPermitida(1);
                controlPos =1;
              state bajarCarro
                entry: vtauto=0;
              state parar
                entry: vhauto=0;
                during:
                if temporalCount(sec) >20
                finOperacion=1;
                end
              (default) -> automata.grua.maquinaOperando.opAutomatica.controlMovimientos.muelleAlBarco.subirIzaje
              automata.grua.maquinaOperando.opAutomatica.controlMovimientos.muelleAlBarco.subirIzaje -> automata.grua.maquinaOperando.opAutomatica.controlMovimientos.muelleAlBarco.subirYdesplazarCarro : [y_actual>=alturaInicioDesplazamientoCarro]
              automata.grua.maquinaOperando.opAutomatica.controlMovimientos.muelleAlBarco.subirYdesplazarCarro -> automata.grua.maquinaOperando.opAutomatica.controlMovimientos.muelleAlBarco.moverCarro : [y_actual>=ySeguridadCarro-cteAlturaSuperior]
              automata.grua.maquinaOperando.opAutomatica.controlMovimientos.muelleAlBarco.moverCarro -> automata.grua.maquinaOperando.opAutomatica.controlMovimientos.muelleAlBarco.bajarYdesplazarCarro : [xt>=PosicionCarroInicioDescensoIzaje-cteDestino]
              automata.grua.maquinaOperando.opAutomatica.controlMovimientos.muelleAlBarco.bajarYdesplazarCarro -> automata.grua.maquinaOperando.opAutomatica.controlMovimientos.muelleAlBarco.bajarCarro : [xt>=x_destino-cteDestino-cteCarro]
              automata.grua.maquinaOperando.opAutomatica.controlMovimientos.muelleAlBarco.bajarCarro -> automata.grua.maquinaOperando.opAutomatica.controlMovimientos.muelleAlBarco.parar : [y_actual<=y_destino+cteAlturaInferior]
            state start
              entry:
              finOperacion=0;
              vtauto=0;
              vhauto=0;
            start -> muelleAlBarco [order 1] : [xt<0 && x_destino>=0 && botonModoAutomatico]
            start -> barcoAlMuelle [order 2] : [xt>=0 && x_destino<0 && botonModoAutomatico]
            muelleAlBarco -> start : [finOperacion]
            barcoAlMuelle -> start : [finOperacion]
            (default) -> start
          state acutalizarParametros [parallel]
            during:
            if lh<22
            if in(gancho.Gcerrado)
            cteAlturaInferior=6;
            cteAlturaSuperior=-2;
            cteDestino=0;
            cteCarro=10;
            else
            cteAlturaInferior=6;
            cteAlturaSuperior=4;
            cteDestino=5;
            cteCarro=10;
            end
            else
            if in(gancho.Gcerrado)
            cteAlturaInferior=9;
            cteAlturaSuperior=-2;
            cteDestino=0;
            cteCarro=12;
            else
            cteAlturaSuperior1=2;
            cteAlturaInferior=6;
            cteAlturaSuperior=4;
            cteDestino=0;
            cteCarro=12;
            end
            end
            settings: executionOrder=2
        state opManual [parallel]
          settings: executionOrder=2
          state Carro [parallel]
            during:
            if palancaCarro==-1  %izquierda
            vtmanual=-vmaxt; %primer valor es la permitida a la izq
            elseif palancaCarro==0
            vtmanual=0;
            elseif palancaCarro==1
            vtmanual=vmaxt; %segundo valor es la permitida a la der
            end
            settings: executionOrder=2
          state Izaje [parallel]
            during:
            if palancaIzaje==1  % boton abajo
            vhmanual=vhPermitida(1);
            elseif palancaIzaje==0
            vhmanual=0;
            elseif palancaIzaje==-1
            vhmanual=-vhPermitida(2);
            end
            settings: executionOrder=1
      (default) -> maquinaEspera
      maquinaEspera -> maquinaOperando : [botonOperarMaq]
      maquinaOperando -> maquinaEspera : [botonPararMaq  || DetenerNivel1]
  data: dir function_input; t function_input; Vtmanual function_input; Vtauto function_input; Vhmanual function_input; Vt function_output; Vhauto function_input; Vh function_output; y2 function_input; y1 function_input; x2 function_input; x1 function_input; x function_input; yRecta function_output; lh input; xt input; ml input; Time input; botonAbrirGancho input; botonCerrarGancho input; Gcierre output; botonOperarMaq input; botonPararMaq input; botonModoAutomatico input; botonModoManual input; palancaCarro input; palancaIzaje input; botonActivaControlAngulo input; botonDesactivaControlAngulo input; l_max_cable parameter; l_min_cable parameter; mlfull parameter; vh output; vmaxhfull parameter; vmaxh parameter; vhPermitida local; vt output; vtPermitida local; vmaxt parameter; tiempoTableroActivo local; longitudSegMaxCable parameter; longitudSegMinCable parameter; vmaxhSobrepeso parameter; x_destino input; y_origen input; y_destino input; ySeguridadCarro input; PosicionCarroInicioDescensoIzaje input; alturaInicioDesplazamientoCarro input; y_actual input; finOperacion local; dt local; time0 local; vhauto local; vhmanual local; vtauto local; vtmanual local; cteAlturaSuperior local; cteDestino local; controlAngulo output; cteAlturaInferior local; controlPos output; DetenerNivel1 input; cteAlturaSuperior1 local; cteCarro local
  function [Vt,Vh]  = Transferencia(dir,t,Vtmanual,Vtauto,Vhmanual,Vhauto):
    | function [Vt,Vh]  = Transferencia(dir,t,Vtmanual,Vtauto,Vhmanual,Vhauto)
    | 
    | m=1/5*dir;
    | if dir==1
    |     y1=0;
    | elseif dir==-1
    |     y1=1;
    | end
    | yRecta1=m*t+y1;
    | yRecta2=1-yRecta1;
    | Vt=yRecta1*Vtauto+yRecta2*Vtmanual;
    | Vh=yRecta1*Vhauto+yRecta2*Vhmanual;
    | 
    | end
  function yRecta =rectaDosPuntos(y2,y1,x2,x1,x):
    | function yRecta =rectaDosPuntos(y2,y1,x2,x1,x)
    | m=(y2-y1)/(x2-x1);
    | yRecta=m*(x-x1)+y1;
    | end
